simulink model "torqueBalancingSOT_logData"  (Simulink 8.8)
settings: Solver=FixedStepDiscrete  StartTime=0.0  StopTime=CONFIG.SIMULATION_TIME  FixedStep=CONFIG.Ts  RelTol=1e-3  EnableMultiTasking=on
InitFcn:
  | cd(fileparts(which(bdroot)));
  | initTorqueBalancingSOT;
undefined symbols (not defined in the file or in its folder): CONFIG, ConstraintsFeetMatrix, DiscIntNeverNeededParam, gain, reg, ROBOT_DOF, sat, sm, upperBoundFeetConstraints, WBT_robotName
libraries: WBToolboxLibrary x69
(part 1 of 2)
settings Model: SuppressorTable=22 serialization::archive 11 0 3 0 0 0 11 0  Creator=marie  LastModifiedBy=marie
settings DataIOCC: LimitDataPoints=off  SaveFormat=Dataset  SignalLoggingSaveFormat=Dataset
settings DebuggingCC: UnderspecifiedInitializationDetection=Simplified  MergeDetectMultiDrivingBlocksExec=error  FcnCallInpInsideContextMsg=error  StateNameClashWarn=none  SFUnexpectedBacktrackingDiag=error  SFNoUnconditionalDefaultTransitionDiag=error
settings HardwareCC: ProdBitPerPointer=64  ProdBitPerSizeT=64  ProdBitPerPtrDiffT=64  ProdLargestAtomicFloat=Float  ProdIntDivRoundTo=Zero  ProdEndianess=LittleEndian  ProdWordSize=64  ProdHWDeviceType=Intel->x86-64 (Windows64)
settings ModelReferenceCC: PropagateSignalLabelsOutOfModel=on
settings GRTTargetCC: TargetLangStandard=C99 (ISO)  GeneratePreprocessorConditionals=Use local settings  CombineOutputUpdateFcns=on  GRTInterface=off
settings ConfigComp: CovMetricSettings=dwe  CovHtmlReporting=off  CovSaveCumulativeToWorkspaceVar=off  CovSaveSingleToWorkspaceVar=off  CovExternalEMLEnable=on

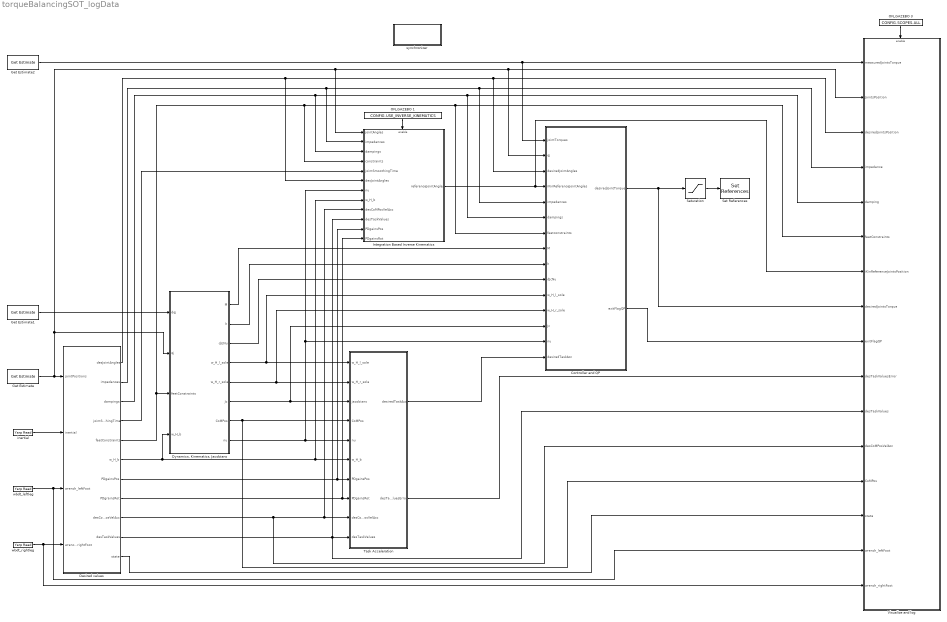
== system torqueBalancingSOT_logData ==
  Controller and QP : Subsystem
  Desired values : Subsystem
  "Dynamics, Kinematics, Jacobians" : Subsystem
  Get Estimate : WBToolboxLibrary/wholeBodyStates/Get Estimate  estimateType=Joints Position  robotName=WBT_robotName  localName=WBT_modelName  wbiFile=WBT_wbiFilename  wbiList=WBT_wbiList
  Get Estimate1 : WBToolboxLibrary/wholeBodyStates/Get Estimate  estimateType=Joints Velocity  robotName=WBT_robotName  localName=WBT_modelName  wbiFile=WBT_wbiFilename  wbiList=WBT_wbiList
  Get Estimate2 : WBToolboxLibrary/wholeBodyStates/Get Estimate  estimateType=Joints Torque  robotName=WBT_robotName  localName=WBT_modelName  wbiFile=WBT_wbiFilename  wbiList=WBT_wbiList
  Integration Based Inverse Kinematics : Subsystem
  ON_GAZEBO 1 : Constant  Value=CONFIG.USE_INVERSE_KINEMATICS
  ON_GAZEBO 3 : Constant  Value=CONFIG.SCOPES.ALL
  Saturation : Saturate  UpperLimit=sat.torque  LowerLimit=-sat.torque
  Set References : WBToolboxLibrary/wholeBodyActuators/Set References  controlType=Torque  fullOrSubControl=Full  controlledJoints=''  robotName=WBT_robotName  localName=WBT_modelName  wbiFile=WBT_wbiFilename  wbiList=WBT_wbiList
  Task Acceleration : Subsystem
  Visualize and log : Subsystem
  inertial : WBToolboxLibrary/Utilities/Yarp Read  portName=PORTS.IMU  signalSize=12  blocking=off  timestamp=off  autoconnect=on  errorOnConnection=on
  synchronizer : Subsystem
      mask Display: disp('SYNCHRONIZER')
  wbdt_leftleg : WBToolboxLibrary/Utilities/Yarp Read  portName=PORTS.WBDT_LEFTLEG_EE  signalSize=6  blocking=off  timestamp=off  autoconnect=on  errorOnConnection=off
  wbdt_rightleg : WBToolboxLibrary/Utilities/Yarp Read  portName=PORTS.WBDT_RIGHTLEG_EE  signalSize=6  blocking=off  timestamp=off  autoconnect=on  errorOnConnection=off
  wires:
  "Dynamics, Kinematics, Jacobians"/7(CoMPos) -> Visualize and log/13(CoMPos), Task Acceleration/4(CoMPos)
  Desired values/9(desCoMPosVelAcc) -> Visualize and log/12(desCoMPosVelAcc), Integration Based Inverse Kinematics/9(desCoMPosVelAcc), Task Acceleration/9(desCoMPosVelAcc)
  "Dynamics, Kinematics, Jacobians"/8(nu) -> Integration Based Inverse Kinematics/7(nu), Controller and QP/14(nu), Task Acceleration/5(nu)
  Desired values/10(desTaskValues) -> Integration Based Inverse Kinematics/10(desTaskValues), Visualize and log/11(desTaskValues), Task Acceleration/10(desTaskValues)
  Desired values/7(PDgainsPos) -> Integration Based Inverse Kinematics/11(PDgainsPos), Task Acceleration/7(PDgainsPos)
  "Dynamics, Kinematics, Jacobians"/5(w_H_r_sole) -> Controller and QP/12(w_H_r_sole), Task Acceleration/2(w_H_r_sole)
  "Dynamics, Kinematics, Jacobians"/4(w_H_l_sole) -> Controller and QP/11(w_H_l_sole), Task Acceleration/1(w_H_l_sole)
  Desired values/2(impedances) -> Integration Based Inverse Kinematics/2(impedances), Visualize and log/4(impedance), Controller and QP/5(impedances)
  "Dynamics, Kinematics, Jacobians"/1(M) -> Controller and QP/8(M)
  "Dynamics, Kinematics, Jacobians"/2(h) -> Controller and QP/9(h)
  Desired values/3(dampings) -> Integration Based Inverse Kinematics/3(dampings), Controller and QP/6(dampings), Visualize and log/5(damping)
  Controller and QP/1(desiredJointTorques) -> Saturation/1, Visualize and log/8(desiredJointsTorque)
  Saturation/1 -> Set References/1
  ON_GAZEBO 3/1 -> Visualize and log/Enable
  Controller and QP/2(exitFlagQP) -> Visualize and log/9(exitFlagQP)
  Task Acceleration/2(desTaskValuesError) -> Visualize and log/10(desTaskValuesError)
  inertial/1 -> Desired values/2(inertial)
  wbdt_leftleg/1 -> Desired values/3(wrench_leftFoot), Visualize and log/15(wrench_leftFoot)
  wbdt_rightleg/1 -> Desired values/4(wrench_rightFoot), Visualize and log/16(wrench_rightFoot)
  Get Estimate1/1 -> "Dynamics, Kinematics, Jacobians"/1(dqj)
  Get Estimate2/1 -> Visualize and log/1(measuredJointsTorque), Controller and QP/1(jointTorques)
  Desired values/6(w_H_b) -> "Dynamics, Kinematics, Jacobians"/4(w_H_b), Integration Based Inverse Kinematics/8(w_H_b), Task Acceleration/6(w_H_b)
  Get Estimate/1 -> Visualize and log/2(JointsPosition), Controller and QP/2(qj), Integration Based Inverse Kinematics/1(jointAngles), "Dynamics, Kinematics, Jacobians"/2(qj), Desired values/1(jointPositions)
  "Dynamics, Kinematics, Jacobians"/6(Jc) -> Controller and QP/13(Jc), Task Acceleration/3(jacobians)
  Desired values/5(feetConstraints) -> Controller and QP/7(feetconstraints), Visualize and log/6(feetConstraints), Integration Based Inverse Kinematics/4(constraints), "Dynamics, Kinematics, Jacobians"/3(feetConstraints)
  "Dynamics, Kinematics, Jacobians"/3(dJcNu) -> Controller and QP/10(dJcNu)
  Task Acceleration/1(desiredTaskAcc) -> Controller and QP/15(desiredTaskAcc)
  Desired values/11(state) -> Visualize and log/14(state)
  Integration Based Inverse Kinematics/1(referenceJointAngles) -> Visualize and log/7(iKinReferenceJointsPosition), Controller and QP/4(iKinReferenceJointAngles)
  Desired values/1(desJointAngles) -> Integration Based Inverse Kinematics/6(desJointAngles), Visualize and log/3(desiredJointsPosition), Controller and QP/3(desiredJointAngles)
  ON_GAZEBO 1/1 -> Integration Based Inverse Kinematics/Enable
  Desired values/8(PDgrainsRot) -> Integration Based Inverse Kinematics/12(PDgainsRot), Task Acceleration/8(PDgainsRot)
  Desired values/4(jointSmoothingTime) -> Integration Based Inverse Kinematics/5(jointSmoothingTime)

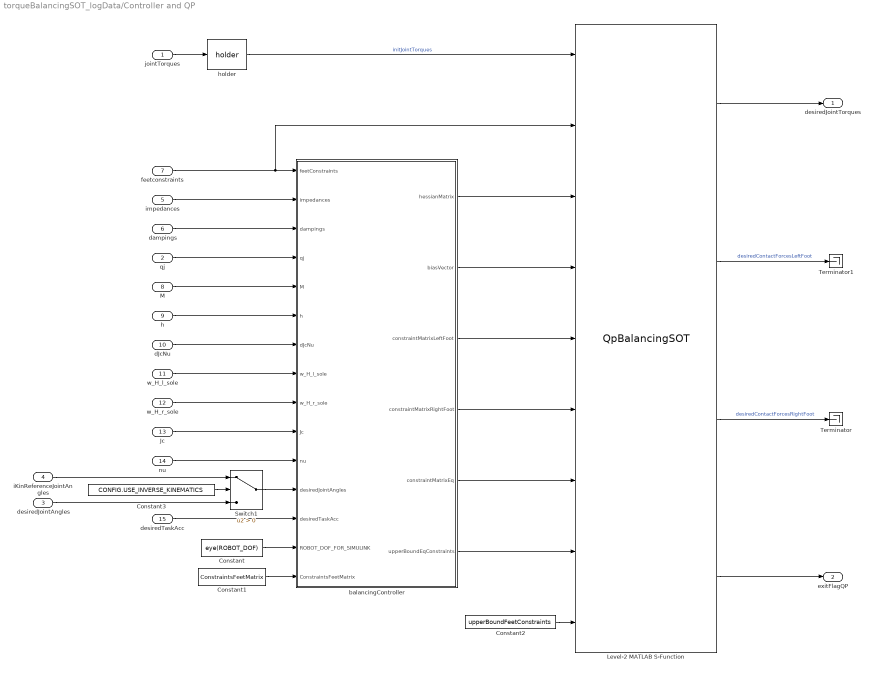
== system torqueBalancingSOT_logData/Controller and QP ==
  jointTorques : Inport
  qj : Inport  Port=2
  desiredJointAngles : Inport  Port=3
  iKinReferenceJointAngles : Inport  Port=4
  impedances : Inport  Port=5
  dampings : Inport  Port=6
  feetconstraints : Inport  Port=7
  M : Inport  Port=8
  h : Inport  Port=9
  dJcNu : Inport  Port=10
  w_H_l_sole : Inport  Port=11
  w_H_r_sole : Inport  Port=12
  Jc : Inport  Port=13
  nu : Inport  Port=14
  desiredTaskAcc : Inport  Port=15
  Constant : Constant  Value=eye(ROBOT_DOF)
  Constant1 : Constant  Value=ConstraintsFeetMatrix
  Constant2 : Constant  Value=upperBoundFeetConstraints
  Constant3 : Constant  Value=CONFIG.USE_INVERSE_KINEMATICS
  Level-2 MATLAB S-Function : M-S-Function  FunctionName=QpBalancingSOT  Parameters=ROBOT_DOF,sat.torqueDot,CONFIG.Ts,CONFIG.QP.USE_CONTINUITY_CONSTRAINTS,CONFIG.QP.USE_STRICT_TASK_PRIORITIES  mask{robotDofs=ROBOT_DOF, tauDotMax=sat.torqueDot, Ts=CONFIG.Ts}
      mask prompts: robotDofs "Robt degrees of freedom"; tauDotMax "Maximum derivative of torques"; Ts "Controller period"
      mask Display: disp('QP')
  Switch1 : Switch  Criteria=u2 > Threshold
  Terminator : Terminator
  Terminator1 : Terminator
  balancingController : MATLAB Function  TreatAsAtomicUnit=on
  "holder " : WBToolboxLibrary/Utilities/holder 
  desiredJointTorques : Outport
  exitFlagQP : Outport  Port=2
  wires:
  balancingController/1(hessianMatrix) -> Level-2 MATLAB S-Function/3
  feetconstraints/1 -> Level-2 MATLAB S-Function/2, balancingController/1(feetConstraints)
  qj/1 -> balancingController/4(qj)
  impedances/1 -> balancingController/2(impedances)
  M/1 -> balancingController/5(M)
  h/1 -> balancingController/6(h)
  dJcNu/1 -> balancingController/7(dJcNu)
  w_H_l_sole/1 -> balancingController/8(w_H_l_sole)
  w_H_r_sole/1 -> balancingController/9(w_H_r_sole)
  Jc/1 -> balancingController/10(Jc)
  nu/1 -> balancingController/11(nu)
  desiredTaskAcc/1 -> balancingController/13(desiredTaskAcc)
  Constant/1 -> balancingController/14(ROBOT_DOF_FOR_SIMULINK)
  Constant1/1 -> balancingController/15(ConstraintsFeetMatrix)
  dampings/1 -> balancingController/3(dampings)
  balancingController/2(biasVector) -> Level-2 MATLAB S-Function/4
  balancingController/3(constraintMatrixLeftFoot) -> Level-2 MATLAB S-Function/5
  balancingController/4(constraintMatrixRightFoot) -> Level-2 MATLAB S-Function/6
  balancingController/5(constraintMatrixEq) -> Level-2 MATLAB S-Function/7
  balancingController/6(upperBoundEqConstraints) -> Level-2 MATLAB S-Function/8
  Constant2/1 -> Level-2 MATLAB S-Function/9
  Level-2 MATLAB S-Function/1 -> desiredJointTorques/1
  Level-2 MATLAB S-Function/2 -> Terminator1/1  "desiredContactForcesLeftFoot"
  Level-2 MATLAB S-Function/3 -> Terminator/1  "desiredContactForcesRightFoot"
  Level-2 MATLAB S-Function/4 -> exitFlagQP/1
  jointTorques/1 -> "holder "/1
  "holder "/1 -> Level-2 MATLAB S-Function/1  "initJointTorques"
  Constant3/1 -> Switch1/2
  iKinReferenceJointAngles/1 -> Switch1/1
  desiredJointAngles/1 -> Switch1/3
  Switch1/1 -> balancingController/12(desiredJointAngles)

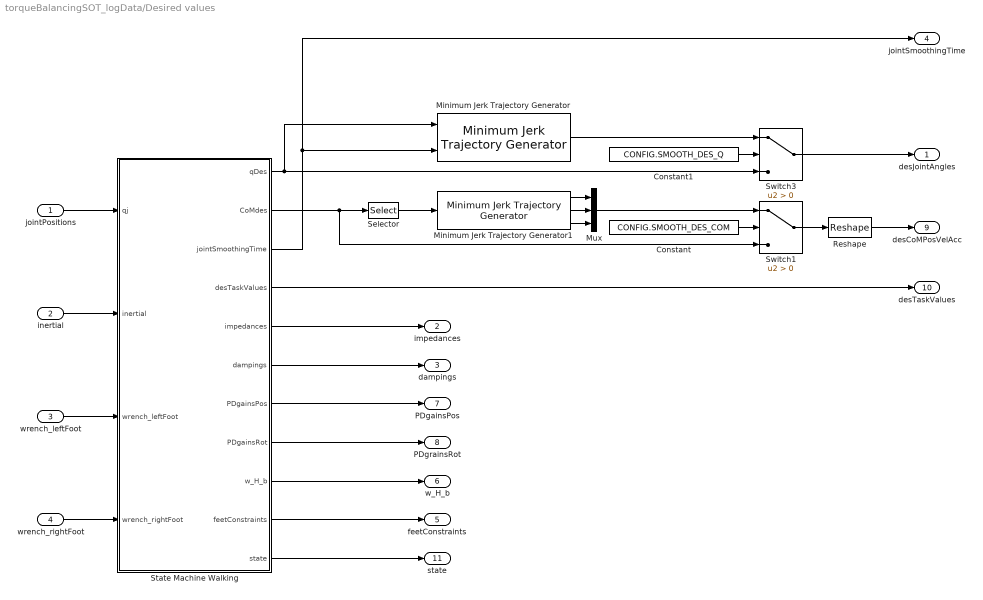
== system torqueBalancingSOT_logData/Desired values ==
  jointPositions : Inport
  inertial : Inport  Port=2
  wrench_leftFoot : Inport  Port=3
  wrench_rightFoot : Inport  Port=4
  Constant : Constant  Value=CONFIG.SMOOTH_DES_COM
  Constant1 : Constant  Value=CONFIG.SMOOTH_DES_Q
  Minimum Jerk Trajectory Generator : WBToolboxLibrary/Utilities/Minimum Jerk Trajectory Generator  externalSettlingTime=on  settlingTime=3  sampleTime=CONFIG.Ts  resetOnSettlingTime=off  firstDerivatives=off  secondDerivatives=off  explicitInitialValue=off
  Minimum Jerk Trajectory Generator1 : WBToolboxLibrary/Utilities/Minimum Jerk Trajectory Generator  externalSettlingTime=off  settlingTime=gain.SmoothingTimeTasks  sampleTime=CONFIG.Ts  resetOnSettlingTime=off  firstDerivatives=on  secondDerivatives=on  explicitInitialValue=off
  Mux : Mux  Inputs=3
  Reshape : Reshape  OutputDimensionality=Customize  OutputDimensions=[3,3]
  Selector : Selector  InputPortWidth=9  IndexOptions=Index vector (dialog)  Indices=[1 2 3]  OutputSizes=1
  State Machine Walking : Subsystem
  Switch1 : Switch  Criteria=u2 > Threshold
  Switch3 : Switch  Criteria=u2 > Threshold
  desJointAngles : Outport
  impedances : Outport  Port=2
  dampings : Outport  Port=3
  jointSmoothingTime : Outport  Port=4
  feetConstraints : Outport  Port=5
  w_H_b : Outport  Port=6
  PDgainsPos : Outport  Port=7
  PDgrainsRot : Outport  Port=8
  desCoMPosVelAcc : Outport  Port=9
  desTaskValues : Outport  Port=10
  state : Outport  Port=11
  wires:
  Constant/1 -> Switch1/2
  Constant1/1 -> Switch3/2
  Minimum Jerk Trajectory Generator1/3 -> Mux/3
  Minimum Jerk Trajectory Generator1/2 -> Mux/2
  State Machine Walking/7(PDgainsPos) -> PDgainsPos/1
  State Machine Walking/9(w_H_b) -> w_H_b/1
  State Machine Walking/11(state) -> state/1
  Mux/1 -> Switch1/1
  Minimum Jerk Trajectory Generator1/1 -> Mux/1
  State Machine Walking/5(impedances) -> impedances/1
  Selector/1 -> Minimum Jerk Trajectory Generator1/1
  State Machine Walking/3(jointSmoothingTime) -> jointSmoothingTime/1, Minimum Jerk Trajectory Generator/2
  Switch1/1 -> Reshape/1
  Switch3/1 -> desJointAngles/1
  State Machine Walking/2(CoMdes) -> Switch1/3, Selector/1
  State Machine Walking/4(desTaskValues) -> desTaskValues/1
  State Machine Walking/10(feetConstraints) -> feetConstraints/1
  State Machine Walking/1(qDes) -> Minimum Jerk Trajectory Generator/1, Switch3/3
  Reshape/1 -> desCoMPosVelAcc/1
  jointPositions/1 -> State Machine Walking/1(qj)
  State Machine Walking/6(dampings) -> dampings/1
  wrench_rightFoot/1 -> State Machine Walking/4(wrench_rightFoot)
  wrench_leftFoot/1 -> State Machine Walking/3(wrench_leftFoot)
  inertial/1 -> State Machine Walking/2(inertial)
  State Machine Walking/8(PDgainsRot) -> PDgrainsRot/1
  Minimum Jerk Trajectory Generator/1 -> Switch3/1

== system torqueBalancingSOT_logData/Dynamics, Kinematics, Jacobians ==
  dqj : Inport
  qj : Inport  Port=2
  feetConstraints : Inport  Port=3
  w_H_b : Inport  Port=4
  CoM/Base Kinematics : Subsystem
  Jacobians : Subsystem
  System Dynamics : Subsystem
  M : Outport
  h : Outport  Port=2
  dJcNu : Outport  Port=3
  w_H_l_sole : Outport  Port=4
  w_H_r_sole : Outport  Port=5
  Jc : Outport  Port=6
  CoMPos : Outport  Port=7
  nu : Outport  Port=8
  wires:
  qj/1 -> Jacobians/4(qj), System Dynamics/3(qj), CoM/Base Kinematics/2(qj)
  w_H_b/1 -> Jacobians/3(w_H_b), System Dynamics/2(w_H_b), CoM/Base Kinematics/1(w_H_b)
  CoM/Base Kinematics/1(CoMPos) -> CoMPos/1
  Jacobians/1(Jc) -> Jc/1
  Jacobians/2(dJcNu) -> dJcNu/1
  System Dynamics/2(M) -> M/1
  System Dynamics/1(h) -> h/1
  CoM/Base Kinematics/2(w_H_l_sole) -> w_H_l_sole/1
  CoM/Base Kinematics/3(w_H_r_sole) -> w_H_r_sole/1
  dqj/1 -> Jacobians/2(dqj)
  feetConstraints/1 -> Jacobians/1(feetConstraints)
  Jacobians/3(nu) -> nu/1, System Dynamics/1(nu)

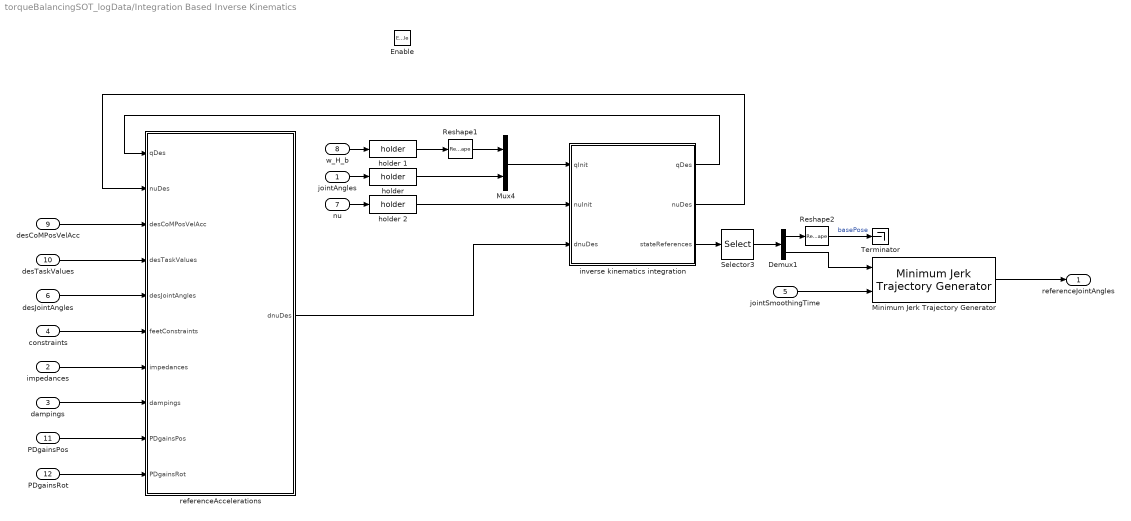
== system torqueBalancingSOT_logData/Integration Based Inverse Kinematics ==
  jointAngles : Inport
  impedances : Inport  Port=2
  dampings : Inport  Port=3
  constraints : Inport  Port=4
  jointSmoothingTime : Inport  Port=5
  desJointAngles : Inport  Port=6
  nu : Inport  Port=7
  w_H_b : Inport  Port=8
  desCoMPosVelAcc : Inport  Port=9
  desTaskValues : Inport  Port=10
  PDgainsPos : Inport  Port=11
  PDgainsRot : Inport  Port=12
  Enable : EnablePort
  Demux1 : Demux  Outputs=[16,ROBOT_DOF]
  Minimum Jerk Trajectory Generator : WBToolboxLibrary/Utilities/Minimum Jerk Trajectory Generator  externalSettlingTime=on  settlingTime=0.5  sampleTime=CONFIG.Ts  resetOnSettlingTime=off  firstDerivatives=off  secondDerivatives=off  explicitInitialValue=off
  Mux4 : Mux  Inputs=2
  Reshape1 : Reshape
  Reshape2 : Reshape  OutputDimensionality=Customize  OutputDimensions=[4,4]
  Selector3 : Selector  NumberOfDimensions=2  InputPortWidth=3  IndexOptions=Index vector (dialog),Index vector (dialog)  Indices=[1:(ROBOT_DOF+16)],[1]  OutputSizes=1,1
  Terminator : Terminator
  "holder " : WBToolboxLibrary/Utilities/holder 
  holder 1 : WBToolboxLibrary/Utilities/holder 
  holder 2 : WBToolboxLibrary/Utilities/holder 
  inverse kinematics integration : Subsystem
  referenceAccelerations : Subsystem
  referenceJointAngles : Outport
  wires:
  Mux4/1 -> inverse kinematics integration/1(qInit)
  desCoMPosVelAcc/1 -> referenceAccelerations/3(desCoMPosVelAcc)
  constraints/1 -> referenceAccelerations/6(feetConstraints)
  holder 1/1 -> Reshape1/1
  Reshape1/1 -> Mux4/1
  "holder "/1 -> Mux4/2
  jointAngles/1 -> "holder "/1
  w_H_b/1 -> holder 1/1
  desJointAngles/1 -> referenceAccelerations/5(desJointAngles)
  desTaskValues/1 -> referenceAccelerations/4(desTaskValues)
  holder 2/1 -> inverse kinematics integration/2(nuInit)
  referenceAccelerations/1(dnuDes) -> inverse kinematics integration/3(dnuDes)
  inverse kinematics integration/1(qDes) -> referenceAccelerations/1(qDes)
  inverse kinematics integration/2(nuDes) -> referenceAccelerations/2(nuDes)
  inverse kinematics integration/3(stateReferences) -> Selector3/1
  nu/1 -> holder 2/1
  Selector3/1 -> Demux1/1
  Reshape2/1 -> Terminator/1  "basePose"
  Demux1/1 -> Reshape2/1
  Demux1/2 -> Minimum Jerk Trajectory Generator/1
  Minimum Jerk Trajectory Generator/1 -> referenceJointAngles/1
  impedances/1 -> referenceAccelerations/7(impedances)
  dampings/1 -> referenceAccelerations/8(dampings)
  PDgainsPos/1 -> referenceAccelerations/9(PDgainsPos)
  PDgainsRot/1 -> referenceAccelerations/10(PDgainsRot)
  jointSmoothingTime/1 -> Minimum Jerk Trajectory Generator/2

== system torqueBalancingSOT_logData/Task Acceleration ==
  w_H_l_sole : Inport
  w_H_r_sole : Inport  Port=2
  jacobians : Inport  Port=3
  CoMPos : Inport  Port=4
  nu : Inport  Port=5
  w_H_b : Inport  Port=6
  PDgainsPos : Inport  Port=7
  PDgainsRot : Inport  Port=8
  desCoMPosVelAcc : Inport  Port=9
  desTaskValues : Inport  Port=10
  Bus Creator : BusCreator  Inputs='rootRotError','leftFootOriginError','leftFootRotError','rightFootOriginError','rightFootRotError'
  Bus Selector : BusSelector  OutputSignals=desRootRotPosVelAcc,desLeftFootOriginPosVelAcc,desLeftFootRotPosVelAcc,desRightFootOriginPosVelAcc,desRightFootRotPosVelAcc
  Product : Product  Multiplication=Matrix(*)
  Reshape : Reshape  OutputDimensionality=Customize  OutputDimensions=[3,2]
  Reshape1 : Reshape  OutputDimensionality=Customize  OutputDimensions=[1,18]
  Selector1 : Selector  NumberOfDimensions=2  InputPortWidth=9  IndexOptions=Index vector (dialog),Index vector (dialog)  Indices=[1:3],[1:3]  OutputSizes=1,1
  desiredTaskAcceleration : MATLAB Function  TreatAsAtomicUnit=on
  desiredTaskAcc : Outport
  desTaskValuesError : Outport  Port=2
  wires:
  Bus Selector/1 -> desiredTaskAcceleration/7(desRootRotPosVelAcc)  "<desRootRotPosVelAcc>"
  Bus Selector/2 -> desiredTaskAcceleration/8(desLeftFootOriginPosVelAcc)  "<desLeftFootOriginPosVelAcc>"
  Bus Selector/3 -> desiredTaskAcceleration/9(desLeftFootRotPosVelAcc)  "<desLeftFootRotPosVelAcc>"
  Bus Selector/4 -> desiredTaskAcceleration/10(desRightFootOriginPosVelAcc)  "<desRightFootOriginPosVelAcc>"
  desTaskValues/1 -> Bus Selector/1
  w_H_b/1 -> Selector1/1
  Bus Selector/5 -> desiredTaskAcceleration/11(desRightFootRotPosVelAcc)  "<desRightFootRotPosVelAcc>"
  jacobians/1 -> Product/1
  nu/1 -> Product/2
  CoMPos/1 -> desiredTaskAcceleration/4(CoMPos)
  desCoMPosVelAcc/1 -> desiredTaskAcceleration/6(desCoMPosVelAcc)
  Product/1 -> desiredTaskAcceleration/3(taskVelocities)
  desiredTaskAcceleration/2(rootRotError) -> Bus Creator/1
  desiredTaskAcceleration/3(leftFootOriginError) -> Bus Creator/2
  desiredTaskAcceleration/4(leftFootRotError) -> Bus Creator/3
  desiredTaskAcceleration/5(rightFootOriginError) -> Bus Creator/4
  desiredTaskAcceleration/6(rightFootRotError) -> Bus Creator/5
  desiredTaskAcceleration/1(desiredTaskAcc) -> desiredTaskAcc/1
  Bus Creator/1 -> desTaskValuesError/1
  w_H_r_sole/1 -> desiredTaskAcceleration/2(w_H_r_sole)
  w_H_l_sole/1 -> desiredTaskAcceleration/1(w_H_l_sole)
  Selector1/1 -> desiredTaskAcceleration/5(fixedLink_R_root)
  PDgainsRot/1 -> Reshape/1
  Reshape/1 -> desiredTaskAcceleration/13(PDgainsRot)
  PDgainsPos/1 -> Reshape1/1
  Reshape1/1 -> desiredTaskAcceleration/12(PDgainsPos)

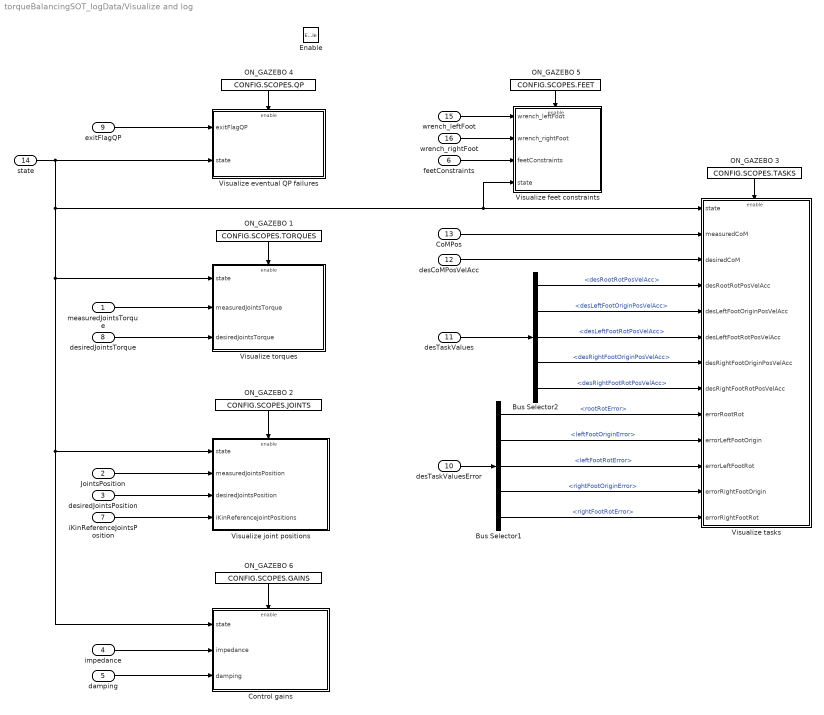
== system torqueBalancingSOT_logData/Visualize and log ==
  measuredJointsTorque : Inport
  JointsPosition : Inport  Port=2
  desiredJointsPosition : Inport  Port=3
  impedance : Inport  Port=4
  damping : Inport  Port=5
  feetConstraints : Inport  Port=6
  iKinReferenceJointsPosition : Inport  Port=7
  desiredJointsTorque : Inport  Port=8
  exitFlagQP : Inport  Port=9
  desTaskValuesError : Inport  Port=10
  desTaskValues : Inport  Port=11
  desCoMPosVelAcc : Inport  Port=12
  CoMPos : Inport  Port=13
  state : Inport  Port=14
  wrench_leftFoot : Inport  Port=15
  wrench_rightFoot : Inport  Port=16
  Enable : EnablePort
  Bus Selector1 : BusSelector  OutputSignals=rootRotError,leftFootOriginError,leftFootRotError,rightFootOriginError,rightFootRotError
  Bus Selector2 : BusSelector  OutputSignals=desRootRotPosVelAcc,desLeftFootOriginPosVelAcc,desLeftFootRotPosVelAcc,desRightFootOriginPosVelAcc,desRightFootRotPosVelAcc
  Control gains : Subsystem
  ON_GAZEBO 1 : Constant  Value=CONFIG.SCOPES.TORQUES
  ON_GAZEBO 2 : Constant  Value=CONFIG.SCOPES.JOINTS
  ON_GAZEBO 3 : Constant  Value=CONFIG.SCOPES.TASKS
  ON_GAZEBO 4 : Constant  Value=CONFIG.SCOPES.QP
  ON_GAZEBO 5 : Constant  Value=CONFIG.SCOPES.FEET
  ON_GAZEBO 6 : Constant  Value=CONFIG.SCOPES.GAINS
  Visualize eventual QP failures : Subsystem
  Visualize feet constraints : Subsystem
  Visualize joint positions : Subsystem
  Visualize tasks : Subsystem
  Visualize torques : Subsystem
  wires:
  ON_GAZEBO 4/1 -> Visualize eventual QP failures/Enable
  exitFlagQP/1 -> Visualize eventual QP failures/1(exitFlagQP)
  measuredJointsTorque/1 -> Visualize torques/2(measuredJointsTorque)
  desiredJointsTorque/1 -> Visualize torques/3(desiredJointsTorque)
  ON_GAZEBO 1/1 -> Visualize torques/Enable
  state/1 -> Visualize eventual QP failures/2(state), Control gains/1(state), Visualize joint positions/1(state), Visualize torques/1(state), Visualize feet constraints/4(state), Visualize tasks/1(state)
  JointsPosition/1 -> Visualize joint positions/2(measuredJointsPosition)
  desiredJointsPosition/1 -> Visualize joint positions/3(desiredJointsPosition)
  ON_GAZEBO 2/1 -> Visualize joint positions/Enable
  CoMPos/1 -> Visualize tasks/2(measuredCoM)
  desCoMPosVelAcc/1 -> Visualize tasks/3(desiredCoM)
  Bus Selector2/3 -> Visualize tasks/6(desLeftFootRotPosVelAcc)  "<desLeftFootRotPosVelAcc>"
  Bus Selector2/2 -> Visualize tasks/5(desLeftFootOriginPosVelAcc)  "<desLeftFootOriginPosVelAcc>"
  Bus Selector2/5 -> Visualize tasks/8(desRightFootRotPosVelAcc)  "<desRightFootRotPosVelAcc>"
  Bus Selector2/4 -> Visualize tasks/7(desRightFootOriginPosVelAcc)  "<desRightFootOriginPosVelAcc>"
  desTaskValues/1 -> Bus Selector2/1
  Bus Selector2/1 -> Visualize tasks/4(desRootRotPosVelAcc)  "<desRootRotPosVelAcc>"
  desTaskValuesError/1 -> Bus Selector1/1
  Bus Selector1/1 -> Visualize tasks/9(errorRootRot)  "<rootRotError>"
  Bus Selector1/2 -> Visualize tasks/10(errorLeftFootOrigin)  "<leftFootOriginError>"
  Bus Selector1/3 -> Visualize tasks/11(errorLeftFootRot)  "<leftFootRotError>"
  Bus Selector1/4 -> Visualize tasks/12(errorRightFootOrigin)  "<rightFootOriginError>"
  Bus Selector1/5 -> Visualize tasks/13(errorRightFootRot)  "<rightFootRotError>"
  ON_GAZEBO 3/1 -> Visualize tasks/Enable
  feetConstraints/1 -> Visualize feet constraints/3(feetConstraints)
  ON_GAZEBO 5/1 -> Visualize feet constraints/Enable
  wrench_rightFoot/1 -> Visualize feet constraints/2(wrench_rightFoot)
  wrench_leftFoot/1 -> Visualize feet constraints/1(wrench_leftFoot)
  impedance/1 -> Control gains/2(impedance)
  damping/1 -> Control gains/3(damping)
  ON_GAZEBO 6/1 -> Control gains/Enable
  iKinReferenceJointsPosition/1 -> Visualize joint positions/4(iKinReferenceJointPositions)

== system torqueBalancingSOT_logData/synchronizer ==
  GAZEBO_SYNCHRONIZER : Subsystem
  Logical Operator : Logic  Operator=NOT  AllPortsSameDT=off  OutDataTypeStr=boolean
  "ON_GAZEBO " : Constant  Value=CONFIG.ON_GAZEBO
  REAL_TIME_SYNC : Subsystem
  wires:
  Logical Operator/1 -> REAL_TIME_SYNC/Enable
  "ON_GAZEBO "/1 -> GAZEBO_SYNCHRONIZER/Enable, Logical Operator/1

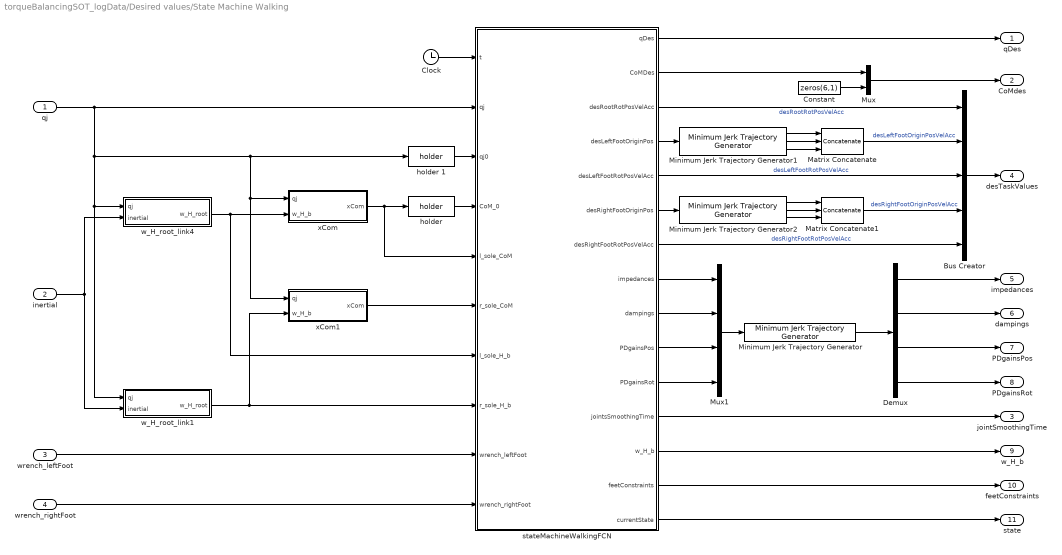
== system torqueBalancingSOT_logData/Desired values/State Machine Walking ==
  qj : Inport
  inertial : Inport  Port=2
  wrench_leftFoot : Inport  Port=3
  wrench_rightFoot : Inport  Port=4
  Bus Creator : BusCreator  Inputs='desRootRotPosVelAcc','desLeftFootOriginPosVelAcc','desLeftFootRotPosVelAcc','desRightFootOriginPosVelAcc','desRightFootRotPosVelAcc'
  Clock : Clock
  Constant : Constant  Value=zeros(6,1)
  Demux : Demux  Outputs=[ROBOT_DOF, ROBOT_DOF, 18, 6]
  Matrix Concatenate : Concatenate  NumInputs=3  Mode=Multidimensional array  ConcatenateDimension=2
  Matrix Concatenate1 : Concatenate  NumInputs=3  Mode=Multidimensional array  ConcatenateDimension=2
  Minimum Jerk Trajectory Generator : WBToolboxLibrary/Utilities/Minimum Jerk Trajectory Generator  externalSettlingTime=off  settlingTime=gain.SmoothingTimeGainScheduling  sampleTime=CONFIG.Ts  resetOnSettlingTime=off  firstDerivatives=off  secondDerivatives=off  explicitInitialValue=off
  Minimum Jerk Trajectory Generator1 : WBToolboxLibrary/Utilities/Minimum Jerk Trajectory Generator  externalSettlingTime=off  settlingTime=gain.SmoothingTimeTasks  sampleTime=CONFIG.Ts  resetOnSettlingTime=off  firstDerivatives=on  secondDerivatives=on  explicitInitialValue=off
  Minimum Jerk Trajectory Generator2 : WBToolboxLibrary/Utilities/Minimum Jerk Trajectory Generator  externalSettlingTime=off  settlingTime=gain.SmoothingTimeTasks  sampleTime=CONFIG.Ts  resetOnSettlingTime=off  firstDerivatives=on  secondDerivatives=on  explicitInitialValue=off
  Mux : Mux  Inputs=2
  Mux1 : Mux
  "holder " : WBToolboxLibrary/Utilities/holder 
  holder 1 : WBToolboxLibrary/Utilities/holder 
  stateMachineWalkingFCN : MATLAB Function  TreatAsAtomicUnit=on
  w_H_root_link1 : Subsystem  mask{link_name='r_sole'}
      mask prompts: link_name "link name"
      mask help:
      | This block evaluates the homogeneous transformation between the world and the root link, i.e. ^wH_b. It assumes that the link specified by the variable 'link_name' has a constant position
      | w.r.t. an inertial frame, but it can rotate arbitrarily. This rotation is retrived from the IMU sensor.
      mask Display:
      | str = strrep(link_name, '_','\_');
      | port_label('output',1,['{}^{',str '}H_{root}'],'texmode','on')
      | clear str;
      | 
      | port_label('input',1,'q_j','texmode','on')
      | 
      | port_label('input',2,'inertial','texmode','on')
  w_H_root_link4 : Subsystem  mask{link_name='l_sole'}
      mask prompts: link_name "link name"
      mask help:
      | This block evaluates the homogeneous transformation between the world and the root link, i.e. ^wH_b. It assumes that the link specified by the variable 'link_name' has a constant position
      | w.r.t. an inertial frame, but it can rotate arbitrarily. This rotation is retrived from the IMU sensor.
      mask Display:
      | str = strrep(link_name, '_','\_');
      | port_label('output',1,['{}^{',str '}H_{root}'],'texmode','on')
      | clear str;
      | 
      | port_label('input',1,'q_j','texmode','on')
      | 
      | port_label('input',2,'inertial','texmode','on')
  xCom : Subsystem
  xCom1 : Subsystem
  qDes : Outport
  CoMdes : Outport  Port=2
  jointSmoothingTime : Outport  Port=3
  desTaskValues : Outport  Port=4
  impedances : Outport  Port=5
  dampings : Outport  Port=6
  PDgainsPos : Outport  Port=7
  PDgainsRot : Outport  Port=8
  w_H_b : Outport  Port=9
  feetConstraints : Outport  Port=10
  state : Outport  Port=11
  wires:
  Clock/1 -> stateMachineWalkingFCN/1(t)
  stateMachineWalkingFCN/8(impedances) -> Mux1/1
  stateMachineWalkingFCN/7(desRightFootRotPosVelAcc) -> Bus Creator/5  "desRightFootRotPosVelAcc"
  Bus Creator/1 -> desTaskValues/1
  wrench_rightFoot/1 -> stateMachineWalkingFCN/10(wrench_rightFoot)
  stateMachineWalkingFCN/13(w_H_b) -> w_H_b/1
  wrench_leftFoot/1 -> stateMachineWalkingFCN/9(wrench_leftFoot)
  Mux1/1 -> Minimum Jerk Trajectory Generator/1
  qj/1 -> w_H_root_link1/1(qj), w_H_root_link4/1(qj), xCom1/1(qj), xCom/1(qj), holder 1/1, stateMachineWalkingFCN/2(qj)
  holder 1/1 -> stateMachineWalkingFCN/3(qj0)
  xCom1/1(xCom) -> stateMachineWalkingFCN/6(r_sole_CoM)
  "holder "/1 -> stateMachineWalkingFCN/4(CoM_0)
  w_H_root_link4/1(w_H_root) -> stateMachineWalkingFCN/7(l_sole_H_b), xCom/2(w_H_b)
  inertial/1 -> w_H_root_link4/2(inertial), w_H_root_link1/2(inertial)
  xCom/1(xCom) -> "holder "/1, stateMachineWalkingFCN/5(l_sole_CoM)
  Minimum Jerk Trajectory Generator/1 -> Demux/1
  stateMachineWalkingFCN/14(feetConstraints) -> feetConstraints/1
  stateMachineWalkingFCN/2(CoMDes) -> Mux/1
  w_H_root_link1/1(w_H_root) -> stateMachineWalkingFCN/8(r_sole_H_b), xCom1/2(w_H_b)
  Demux/1 -> impedances/1
  stateMachineWalkingFCN/12(jointsSmoothingTime) -> jointSmoothingTime/1
  stateMachineWalkingFCN/15(currentState) -> state/1
  stateMachineWalkingFCN/1(qDes) -> qDes/1
  Minimum Jerk Trajectory Generator1/1 -> Matrix Concatenate/1
  Minimum Jerk Trajectory Generator1/2 -> Matrix Concatenate/2
  Minimum Jerk Trajectory Generator1/3 -> Matrix Concatenate/3
  Matrix Concatenate/1 -> Bus Creator/2  "desLeftFootOriginPosVelAcc"
  stateMachineWalkingFCN/4(desLeftFootOriginPos) -> Minimum Jerk Trajectory Generator1/1
  Minimum Jerk Trajectory Generator2/1 -> Matrix Concatenate1/1
  Minimum Jerk Trajectory Generator2/2 -> Matrix Concatenate1/2
  Minimum Jerk Trajectory Generator2/3 -> Matrix Concatenate1/3
  stateMachineWalkingFCN/6(desRightFootOriginPos) -> Minimum Jerk Trajectory Generator2/1
  Matrix Concatenate1/1 -> Bus Creator/4  "desRightFootOriginPosVelAcc"
  stateMachineWalkingFCN/3(desRootRotPosVelAcc) -> Bus Creator/1  "desRootRotPosVelAcc"
  stateMachineWalkingFCN/5(desLeftFootRotPosVelAcc) -> Bus Creator/3  "desLeftFootRotPosVelAcc"
  Demux/3 -> PDgainsPos/1
  Constant/1 -> Mux/2
  Mux/1 -> CoMdes/1
  stateMachineWalkingFCN/9(dampings) -> Mux1/2
  Demux/2 -> dampings/1
  stateMachineWalkingFCN/11(PDgainsRot) -> Mux1/4
  Demux/4 -> PDgainsRot/1
  stateMachineWalkingFCN/10(PDgainsPos) -> Mux1/3

== system torqueBalancingSOT_logData/Dynamics, Kinematics, Jacobians/CoM/Base Kinematics ==
  w_H_b : Inport
  qj : Inport  Port=2
  Forward Kinematics : WBToolboxLibrary/wholeBodyModel/Kinematics/Forward Kinematics  frameName='com'  robotName=WBT_robotName  localName=WBT_modelName  wbiFile=WBT_wbiFilename  wbiList=WBT_wbiList
  Forward Kinematics1 : WBToolboxLibrary/wholeBodyModel/Kinematics/Forward Kinematics  frameName='l_sole'  robotName=WBT_robotName  localName=WBT_modelName  wbiFile=WBT_wbiFilename  wbiList=WBT_wbiList
  Forward Kinematics2 : WBToolboxLibrary/wholeBodyModel/Kinematics/Forward Kinematics  frameName='r_sole'  robotName=WBT_robotName  localName=WBT_modelName  wbiFile=WBT_wbiFilename  wbiList=WBT_wbiList
  Selector : Selector  NumberOfDimensions=2  InputPortWidth=6+ROBOT_DOF  IndexOptions=Index vector (dialog),Index vector (dialog)  Indices=[1:3],[4]  OutputSizes=1,1
  CoMPos : Outport
  w_H_l_sole : Outport  Port=2
  w_H_r_sole : Outport  Port=3
  wires:
  Selector/1 -> CoMPos/1
  qj/1 -> Forward Kinematics1/2, Forward Kinematics2/2, Forward Kinematics/2
  Forward Kinematics/1 -> Selector/1
  w_H_b/1 -> Forward Kinematics1/1, Forward Kinematics2/1, Forward Kinematics/1
  Forward Kinematics2/1 -> w_H_r_sole/1
  Forward Kinematics1/1 -> w_H_l_sole/1

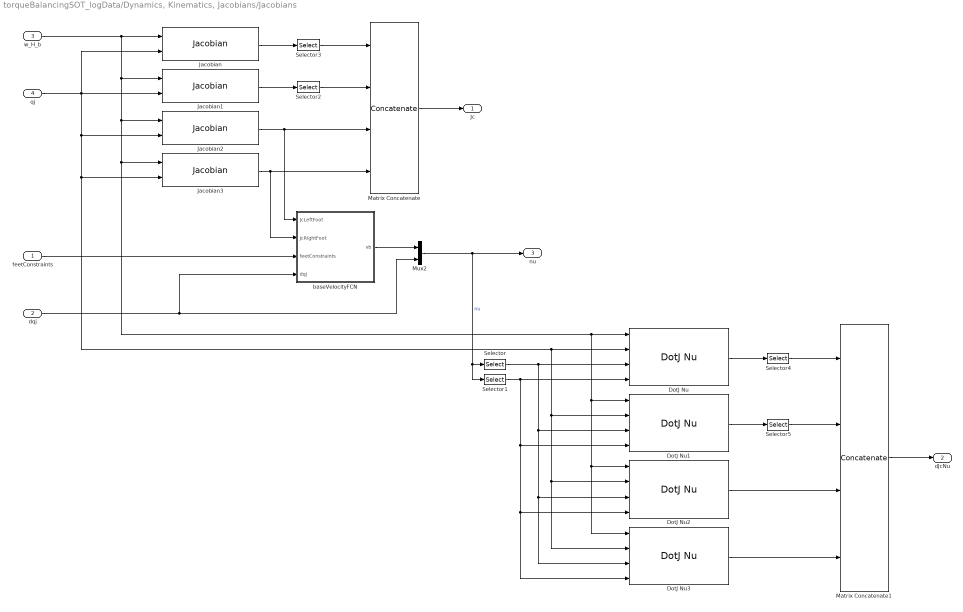
== system torqueBalancingSOT_logData/Dynamics, Kinematics, Jacobians/Jacobians ==
  feetConstraints : Inport
  dqj : Inport  Port=2
  w_H_b : Inport  Port=3
  qj : Inport  Port=4
  DotJ Nu : WBToolboxLibrary/wholeBodyModel/Jacobians/DotJ Nu  frameName='com'  robotName=WBT_robotName  localName=WBT_modelName  wbiFile=WBT_wbiFilename  wbiList=WBT_wbiList
  DotJ Nu1 : WBToolboxLibrary/wholeBodyModel/Jacobians/DotJ Nu  frameName='root_link'  robotName=WBT_robotName  localName=WBT_modelName  wbiFile=WBT_wbiFilename  wbiList=WBT_wbiList
  DotJ Nu2 : WBToolboxLibrary/wholeBodyModel/Jacobians/DotJ Nu  frameName='l_sole'  robotName=WBT_robotName  localName=WBT_modelName  wbiFile=WBT_wbiFilename  wbiList=WBT_wbiList
  DotJ Nu3 : WBToolboxLibrary/wholeBodyModel/Jacobians/DotJ Nu  frameName='r_sole'  robotName=WBT_robotName  localName=WBT_modelName  wbiFile=WBT_wbiFilename  wbiList=WBT_wbiList
  Jacobian : WBToolboxLibrary/wholeBodyModel/Jacobians/Jacobian  frameName='com'  robotName=WBT_robotName  localName=WBT_modelName  wbiFile=WBT_wbiFilename  wbiList=WBT_wbiList
  Jacobian1 : WBToolboxLibrary/wholeBodyModel/Jacobians/Jacobian  frameName='root_link'  robotName=WBT_robotName  localName=WBT_modelName  wbiFile=WBT_wbiFilename  wbiList=WBT_wbiList
  Jacobian2 : WBToolboxLibrary/wholeBodyModel/Jacobians/Jacobian  frameName='l_sole'  robotName=WBT_robotName  localName=WBT_modelName  wbiFile=WBT_wbiFilename  wbiList=WBT_wbiList
  Jacobian3 : WBToolboxLibrary/wholeBodyModel/Jacobians/Jacobian  frameName='r_sole'  robotName=WBT_robotName  localName=WBT_modelName  wbiFile=WBT_wbiFilename  wbiList=WBT_wbiList
  Matrix Concatenate : Concatenate  NumInputs=4  Mode=Multidimensional array
  Matrix Concatenate1 : Concatenate  NumInputs=4  Mode=Multidimensional array
  Mux2 : Mux  Inputs=2
  Selector : Selector  InputPortWidth=6+ROBOT_DOF  IndexOptions=Index vector (dialog)  Indices=[1:6]  OutputSizes=1
  Selector1 : Selector  InputPortWidth=6+ROBOT_DOF  IndexOptions=Index vector (dialog)  Indices=[7:6+ROBOT_DOF]  OutputSizes=1
  Selector2 : Selector  NumberOfDimensions=2  InputPortWidth=6+ROBOT_DOF  IndexOptions=Index vector (dialog),Index vector (dialog)  Indices=[4:6],[1:6+ROBOT_DOF]  OutputSizes=1,1
  Selector3 : Selector  NumberOfDimensions=2  InputPortWidth=6+ROBOT_DOF  IndexOptions=Index vector (dialog),Index vector (dialog)  Indices=[1:3],[1:6+ROBOT_DOF]  OutputSizes=1,1
  Selector4 : Selector  InputPortWidth=6  IndexOptions=Index vector (dialog)  Indices=[1:3]  OutputSizes=1
  Selector5 : Selector  InputPortWidth=6  IndexOptions=Index vector (dialog)  Indices=[4:6]  OutputSizes=1
  baseVelocityFCN : MATLAB Function  TreatAsAtomicUnit=on
  Jc : Outport
  dJcNu : Outport  Port=2
  nu : Outport  Port=3
  wires:
  w_H_b/1 -> DotJ Nu1/1, DotJ Nu3/1, DotJ Nu2/1, DotJ Nu/1, Jacobian3/1, Jacobian2/1, Jacobian1/1, Jacobian/1
  qj/1 -> DotJ Nu3/2, DotJ Nu2/2, DotJ Nu1/2, DotJ Nu/2, Jacobian3/2, Jacobian2/2, Jacobian/2, Jacobian1/2
  Selector/1 -> DotJ Nu3/3, DotJ Nu2/3, DotJ Nu1/3, DotJ Nu/3
  Selector1/1 -> DotJ Nu1/4, DotJ Nu2/4, DotJ Nu3/4, DotJ Nu/4
  Mux2/1 -> nu/1, Selector1/1, Selector/1  "nu"
  Jacobian/1 -> Selector3/1
  Jacobian1/1 -> Selector2/1
  Selector3/1 -> Matrix Concatenate/1
  Selector2/1 -> Matrix Concatenate/2
  Matrix Concatenate/1 -> Jc/1
  DotJ Nu/1 -> Selector4/1
  DotJ Nu1/1 -> Selector5/1
  Selector4/1 -> Matrix Concatenate1/1
  Selector5/1 -> Matrix Concatenate1/2
  DotJ Nu2/1 -> Matrix Concatenate1/3
  DotJ Nu3/1 -> Matrix Concatenate1/4
  Matrix Concatenate1/1 -> dJcNu/1
  Jacobian3/1 -> baseVelocityFCN/2(JcRightFoot), Matrix Concatenate/4
  dqj/1 -> baseVelocityFCN/4(dqj), Mux2/2
  baseVelocityFCN/1(vb) -> Mux2/1
  feetConstraints/1 -> baseVelocityFCN/3(feetConstraints)
  Jacobian2/1 -> Matrix Concatenate/3, baseVelocityFCN/1(JcLeftFoot)

== system torqueBalancingSOT_logData/Dynamics, Kinematics, Jacobians/System Dynamics ==
  nu : Inport
  w_H_b : Inport  Port=2
  qj : Inport  Port=3
  Get Bias Forces : WBToolboxLibrary/wholeBodyModel/Dynamics/Get Bias Forces  robotName=WBT_robotName  localName=WBT_modelName  wbiFile=WBT_wbiFilename  wbiList=WBT_wbiList  explicitGravity=off
  Mass Matrix : WBToolboxLibrary/wholeBodyModel/Dynamics/Mass Matrix  robotName=WBT_robotName  localName=WBT_modelName  wbiFile=WBT_wbiFilename  wbiList=WBT_wbiList
  Selector : Selector  InputPortWidth=6+ROBOT_DOF  IndexOptions=Index vector (dialog)  Indices=[1:6]  OutputSizes=1
  Selector1 : Selector  InputPortWidth=6+ROBOT_DOF  IndexOptions=Index vector (dialog)  Indices=[7:6+ROBOT_DOF]  OutputSizes=1
  h : Outport
  M : Outport  Port=2
  wires:
  Selector/1 -> Get Bias Forces/3
  Selector1/1 -> Get Bias Forces/4
  w_H_b/1 -> Get Bias Forces/1, Mass Matrix/1
  Get Bias Forces/1 -> h/1
  Mass Matrix/1 -> M/1
  qj/1 -> Get Bias Forces/2, Mass Matrix/2
  nu/1 -> Selector1/1, Selector/1

== system torqueBalancingSOT_logData/Integration Based Inverse Kinematics/inverse kinematics integration ==
  qInit : Inport
  nuInit : Inport  Port=2
  dnuDes : Inport  Port=3
  Acceleration Integration : DiscreteIntegrator  InitialConditionSource=external  SampleTime=CONFIG.Ts  ICPrevOutput=DiscIntNeverNeededParam  ICPrevScaledInput=DiscIntNeverNeededParam
  Constant2 : Constant  Value=zeros(10,1)
  Constant3 : Constant  Value=zeros(10,1)
  Demux2 : Demux  Outputs=[7;ROBOT_DOF]
  Demux3 : Demux  Outputs=[6;ROBOT_DOF]
  Matrix Concatenate : Concatenate  NumInputs=3  Mode=Multidimensional array  ConcatenateDimension=2
  Mux3 : Mux  Inputs=2
  Mux4 : Mux  Inputs=2
  Mux5 : Mux  Inputs=2
  Terminator1 : Terminator
  Velocity Integration : DiscreteIntegrator  InitialConditionSource=external  SampleTime=CONFIG.Ts  ICPrevOutput=DiscIntNeverNeededParam  ICPrevScaledInput=DiscIntNeverNeededParam
  baseDerivative : MATLAB Function  TreatAsAtomicUnit=on
  rewrite the base pose as pos+quat : MATLAB Function  TreatAsAtomicUnit=on
  rewrite the base pose as transformation matrix : MATLAB Function  TreatAsAtomicUnit=on
  qDes : Outport
  nuDes : Outport  Port=2
  stateReferences : Outport  Port=3
  wires:
  nuInit/1 -> Acceleration Integration/2
  qInit/1 -> rewrite the base pose as pos+quat/1(qInitQuat)
  dnuDes/1 -> Mux5/2, Acceleration Integration/1
  Demux2/2 -> Terminator1/1
  Demux2/1 -> baseDerivative/1(basePose)
  Velocity Integration/1 -> Demux2/1, rewrite the base pose as transformation matrix/1(qDesQuat)
  Acceleration Integration/1 -> Mux4/2, Demux3/1, nuDes/1
  Demux3/1 -> baseDerivative/2(nuDes_base)
  baseDerivative/1(baseDer) -> Mux3/1
  Demux3/2 -> Mux3/2
  Mux3/1 -> Velocity Integration/1
  Matrix Concatenate/1 -> stateReferences/1
  rewrite the base pose as transformation matrix/1(qDes) -> Matrix Concatenate/1, qDes/1
  rewrite the base pose as pos+quat/1(qInit) -> Velocity Integration/2
  Constant2/1 -> Mux4/1
  Mux4/1 -> Matrix Concatenate/2
  Constant3/1 -> Mux5/1
  Mux5/1 -> Matrix Concatenate/3

== system torqueBalancingSOT_logData/Integration Based Inverse Kinematics/referenceAccelerations ==
  qDes : Inport
  nuDes : Inport  Port=2
  desCoMPosVelAcc : Inport  Port=3
  desTaskValues : Inport  Port=4
  desJointAngles : Inport  Port=5
  feetConstraints : Inport  Port=6
  impedances : Inport  Port=7
  dampings : Inport  Port=8
  PDgainsPos : Inport  Port=9
  PDgainsRot : Inport  Port=10
  Demux : Demux  Outputs=[16;ROBOT_DOF]
  Demux1 : Demux  Outputs=[6;ROBOT_DOF]
  Jacobians : Subsystem
  Kinematics : Subsystem
  Reshape : Reshape  OutputDimensionality=Customize  OutputDimensions=[4,4]
  Task and Joint Accelerations : Subsystem
  trajectoryGeneratorCoM2 : MATLAB Function  TreatAsAtomicUnit=on
  dnuDes : Outport
  wires:
  Demux/1 -> Reshape/1
  Demux1/2 -> Jacobians/4(jointVelocity), Task and Joint Accelerations/2(jointVelocities)
  qDes/1 -> Demux/1
  Reshape/1 -> Kinematics/1(w_H_b), Jacobians/1(w_H_b)
  Demux/2 -> Kinematics/2(JointAngles), Task and Joint Accelerations/4(jointAngles), Jacobians/2(JointAngles)
  feetConstraints/1 -> trajectoryGeneratorCoM2/5(constraints)
  trajectoryGeneratorCoM2/1(dnuDes) -> dnuDes/1
  nuDes/1 -> Demux1/1, Task and Joint Accelerations/3(nuDes)
  Jacobians/1(Jtask) -> Task and Joint Accelerations/1(Jtask), trajectoryGeneratorCoM2/1(Jtask)
  Jacobians/2(dJNu_task) -> trajectoryGeneratorCoM2/2(dJnuDes)
  Demux1/1 -> Jacobians/3(baseVelocity)
  desJointAngles/1 -> Task and Joint Accelerations/5(desJointAngles)
  Kinematics/3(w_H_lsole) -> Task and Joint Accelerations/8(w_H_lsole)
  Kinematics/4(w_H_rsole) -> Task and Joint Accelerations/9(w_H_rsole)
  Kinematics/1(CoMPos) -> Task and Joint Accelerations/6(CoMPos)
  Kinematics/2(w_R_root) -> Task and Joint Accelerations/7(W_R_root)
  desCoMPosVelAcc/1 -> Task and Joint Accelerations/10(desCoMPosVelAcc)
  desTaskValues/1 -> Task and Joint Accelerations/11(desTaskValues)
  Task and Joint Accelerations/2(jointsAccelerations) -> trajectoryGeneratorCoM2/4(jointDynamics)
  Task and Joint Accelerations/1(desTaskAcc) -> trajectoryGeneratorCoM2/3(taskAccelerations)
  impedances/1 -> Task and Joint Accelerations/12(impedances)
  dampings/1 -> Task and Joint Accelerations/13(dampings)
  PDgainsPos/1 -> Task and Joint Accelerations/14(PDgainsPos)
  PDgainsRot/1 -> Task and Joint Accelerations/15(PDgainsRot)

== system torqueBalancingSOT_logData/Visualize and log/Control gains ==
  state : Inport
  impedance : Inport  Port=2
  damping : Inport  Port=3
  Enable : EnablePort
  DoFs converter : WBToolboxLibrary/Utilities/DoFs converter  yarp2WBIOption=From WBI to YARP  robotName=WBT_robotName  localName=WBT_modelName  wbiFile=WBT_wbiFilename  wbiList=WBT_wbiList
  DoFs converter1 : WBToolboxLibrary/Utilities/DoFs converter  yarp2WBIOption=From WBI to YARP  robotName=WBT_robotName  localName=WBT_modelName  wbiFile=WBT_wbiFilename  wbiList=WBT_wbiList
  dampings : Scope  NumInputPorts=6
  impedances : Scope  NumInputPorts=6
  wires:
  DoFs converter/4 -> impedances/4  "left_leg"
  DoFs converter/5 -> impedances/5  "right_leg"
  DoFs converter/1 -> impedances/1  "torso"
  state/1 -> dampings/6, impedances/6  "state"
  DoFs converter1/3 -> dampings/3  "right_arm"
  damping/1 -> DoFs converter1/1
  impedance/1 -> DoFs converter/1
  DoFs converter1/1 -> dampings/1  "torso"
  DoFs converter/2 -> impedances/2  "left_arm"
  DoFs converter1/5 -> dampings/5  "right_leg"
  DoFs converter/3 -> impedances/3  "right_arm"
  DoFs converter1/2 -> dampings/2  "left_arm"
  DoFs converter1/4 -> dampings/4  "left_leg"

== system torqueBalancingSOT_logData/Visualize and log/Visualize eventual QP failures ==
  exitFlagQP : Inport
  state : Inport  Port=2
  Enable : EnablePort
  "QP status (0: no failure,  1: not using,  -1 internal error,  -2:  infeasible, -3:  unbounded) " : Scope  NumInputPorts=2
  wires:
  exitFlagQP/1 -> "QP status (0: no failure,  1: not using,  -1 internal error,  -2:  infeasible, -3:  unbounded) "/1  "exitFlagQP"
  state/1 -> "QP status (0: no failure,  1: not using,  -1 internal error,  -2:  infeasible, -3:  unbounded) "/2

== system torqueBalancingSOT_logData/Visualize and log/Visualize feet constraints ==
  wrench_leftFoot : Inport
  wrench_rightFoot : Inport  Port=2
  feetConstraints : Inport  Port=3
  state : Inport  Port=4
  Enable : EnablePort
  Feet Constraints : Scope  NumInputPorts=4
  wires:
  state/1 -> Feet Constraints/4  "state"
  feetConstraints/1 -> Feet Constraints/3  "feetConstraints"
  wrench_rightFoot/1 -> Feet Constraints/2  "wrench_rightFoot"
  wrench_leftFoot/1 -> Feet Constraints/1  "wrench_leftFoot"

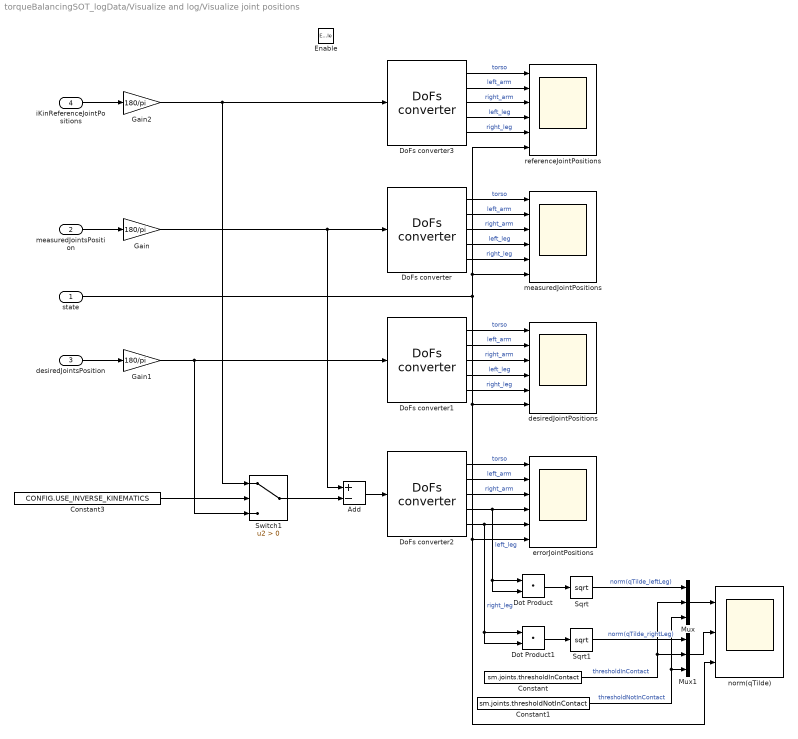
== system torqueBalancingSOT_logData/Visualize and log/Visualize joint positions ==
  state : Inport
  measuredJointsPosition : Inport  Port=2
  desiredJointsPosition : Inport  Port=3
  iKinReferenceJointPositions : Inport  Port=4
  Enable : EnablePort
  Add : Sum  Inputs=+-
  Constant : Constant  Value=sm.joints.thresholdInContact
  Constant1 : Constant  Value=sm.joints.thresholdNotInContact
  Constant3 : Constant  Value=CONFIG.USE_INVERSE_KINEMATICS
  DoFs converter{,1..3} (4 alike) : WBToolboxLibrary/Utilities/DoFs converter  yarp2WBIOption=From WBI to YARP  robotName=WBT_robotName  localName=WBT_modelName  wbiFile=WBT_wbiFilename  wbiList=WBT_wbiList
  Dot Product : DotProduct  InputSameDT=on  OutDataTypeStr=Inherit: Inherit via internal rule
  Dot Product1 : DotProduct  InputSameDT=on  OutDataTypeStr=Inherit: Inherit via internal rule
  Gain : Gain  Gain=180/pi
  Gain1 : Gain  Gain=180/pi
  Gain2 : Gain  Gain=180/pi
  Mux : Mux  Inputs=3
  Mux1 : Mux  Inputs=3
  Sqrt : Sqrt  SaturateOnIntegerOverflow=on
  Sqrt1 : Sqrt  SaturateOnIntegerOverflow=on
  Switch1 : Switch  Criteria=u2 > Threshold
  desiredJointPositions : Scope  NumInputPorts=6
  errorJointPositions : Scope  NumInputPorts=6
  measuredJointPositions : Scope  NumInputPorts=6
  norm(qTilde) : Scope  NumInputPorts=3
  referenceJointPositions : Scope  NumInputPorts=6
  wires:
  DoFs converter/5 -> measuredJointPositions/5  "right_leg"
  DoFs converter/4 -> measuredJointPositions/4  "left_leg"
  DoFs converter/2 -> measuredJointPositions/2  "left_arm"
  DoFs converter/1 -> measuredJointPositions/1  "torso"
  DoFs converter2/2 -> errorJointPositions/2  "left_arm"
  Gain1/1 -> DoFs converter1/1, Switch1/3
  DoFs converter2/1 -> errorJointPositions/1  "torso"
  desiredJointsPosition/1 -> Gain1/1
  measuredJointsPosition/1 -> Gain/1
  DoFs converter2/4 -> errorJointPositions/4, Dot Product/1, Dot Product/2  "left_leg"
  DoFs converter1/1 -> desiredJointPositions/1  "torso"
  DoFs converter1/3 -> desiredJointPositions/3  "right_arm"
  DoFs converter1/4 -> desiredJointPositions/4  "left_leg"
  Add/1 -> DoFs converter2/1
  Gain/1 -> Add/1, DoFs converter/1
  DoFs converter/3 -> measuredJointPositions/3  "right_arm"
  DoFs converter1/2 -> desiredJointPositions/2  "left_arm"
  DoFs converter2/3 -> errorJointPositions/3  "right_arm"
  DoFs converter2/5 -> errorJointPositions/5, Dot Product1/2, Dot Product1/1  "right_leg"
  DoFs converter1/5 -> desiredJointPositions/5  "right_leg"
  state/1 -> referenceJointPositions/6, measuredJointPositions/6, norm(qTilde)/3, errorJointPositions/6, desiredJointPositions/6
  Dot Product/1 -> Sqrt/1
  Dot Product1/1 -> Sqrt1/1
  Sqrt/1 -> Mux/1  "norm(qTilde_leftLeg)"
  Sqrt1/1 -> Mux1/1  "norm(qTilde_rightLeg)"
  Constant/1 -> Mux/2, Mux1/2  "thresholdInContact"
  Constant1/1 -> Mux1/3, Mux/3  "thresholdNotInContact"
  Mux/1 -> norm(qTilde)/1
  Mux1/1 -> norm(qTilde)/2
  DoFs converter3/5 -> referenceJointPositions/5  "right_leg"
  DoFs converter3/4 -> referenceJointPositions/4  "left_leg"
  DoFs converter3/2 -> referenceJointPositions/2  "left_arm"
  DoFs converter3/1 -> referenceJointPositions/1  "torso"
  DoFs converter3/3 -> referenceJointPositions/3  "right_arm"
  iKinReferenceJointPositions/1 -> Gain2/1
  Gain2/1 -> DoFs converter3/1, Switch1/1
  Switch1/1 -> Add/2
  Constant3/1 -> Switch1/2

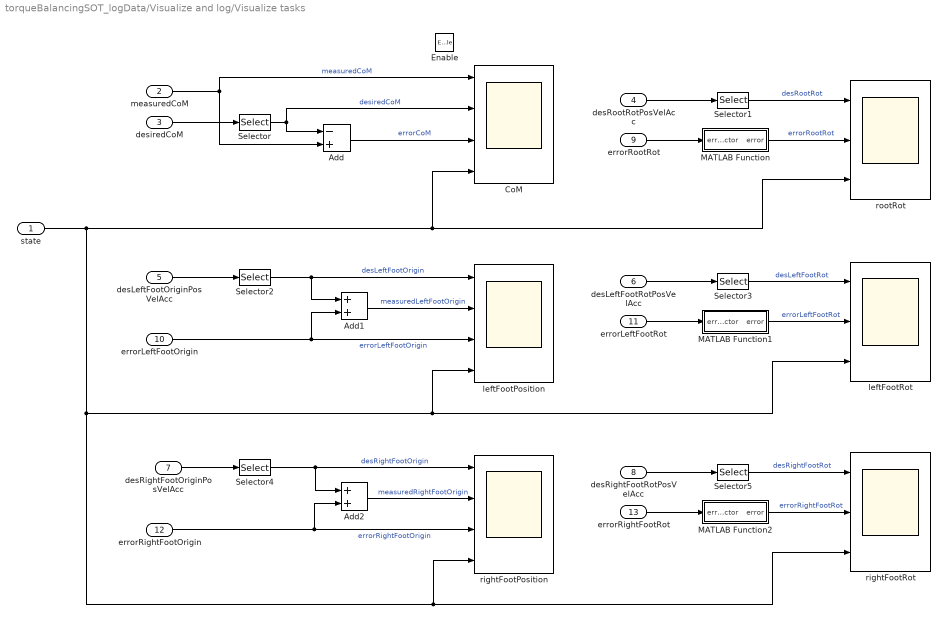
== system torqueBalancingSOT_logData/Visualize and log/Visualize tasks ==
  state : Inport
  measuredCoM : Inport  Port=2
  desiredCoM : Inport  Port=3
  desRootRotPosVelAcc : Inport  Port=4
  desLeftFootOriginPosVelAcc : Inport  Port=5
  desLeftFootRotPosVelAcc : Inport  Port=6
  desRightFootOriginPosVelAcc : Inport  Port=7
  desRightFootRotPosVelAcc : Inport  Port=8
  errorRootRot : Inport  Port=9
  errorLeftFootOrigin : Inport  Port=10
  errorLeftFootRot : Inport  Port=11
  errorRightFootOrigin : Inport  Port=12
  errorRightFootRot : Inport  Port=13
  Enable : EnablePort
  Add : Sum  Inputs=-+
  Add1 : Sum
  Add2 : Sum
  CoM : Scope  NumInputPorts=4
  MATLAB Function : MATLAB Function  TreatAsAtomicUnit=on
  MATLAB Function1 : MATLAB Function  TreatAsAtomicUnit=on
  MATLAB Function2 : MATLAB Function  TreatAsAtomicUnit=on
  Selector : Selector  NumberOfDimensions=2  InputPortWidth=9  IndexOptions=Index vector (dialog),Index vector (dialog)  Indices=[1:3],1  OutputSizes=1,1
  Selector1 : Selector  NumberOfDimensions=2  InputPortWidth=9  IndexOptions=Index vector (dialog),Index vector (dialog)  Indices=[1:3],[1:3]  OutputSizes=1,1
  Selector2 : Selector  NumberOfDimensions=2  InputPortWidth=9  IndexOptions=Index vector (dialog),Index vector (dialog)  Indices=[1:3],1  OutputSizes=1,1
  Selector3 : Selector  NumberOfDimensions=2  InputPortWidth=9  IndexOptions=Index vector (dialog),Index vector (dialog)  Indices=[1:3],[1:3]  OutputSizes=1,1
  Selector4 : Selector  NumberOfDimensions=2  InputPortWidth=9  IndexOptions=Index vector (dialog),Index vector (dialog)  Indices=[1:3],1  OutputSizes=1,1
  Selector5 : Selector  NumberOfDimensions=2  InputPortWidth=9  IndexOptions=Index vector (dialog),Index vector (dialog)  Indices=[1:3],[1:3]  OutputSizes=1,1
  leftFootPosition : Scope  NumInputPorts=4
  leftFootRot : Scope  NumInputPorts=3
  rightFootPosition : Scope  NumInputPorts=4
  rightFootRot : Scope  NumInputPorts=3
  rootRot : Scope  NumInputPorts=3
  wires:
  Selector/1 -> Add/1, CoM/2  "desiredCoM"
  Add/1 -> CoM/3  "errorCoM"
  desiredCoM/1 -> Selector/1
  state/1 -> rootRot/3, CoM/4, rightFootRot/3, rightFootPosition/4, leftFootPosition/4, leftFootRot/3
  measuredCoM/1 -> Add/2, CoM/1  "measuredCoM"
  desLeftFootOriginPosVelAcc/1 -> Selector2/1
  desRightFootOriginPosVelAcc/1 -> Selector4/1
  errorLeftFootOrigin/1 -> Add1/2, leftFootPosition/3  "errorLeftFootOrigin"
  errorRightFootOrigin/1 -> Add2/2, rightFootPosition/3  "errorRightFootOrigin"
  Selector2/1 -> Add1/1, leftFootPosition/1  "desLeftFootOrigin"
  Add1/1 -> leftFootPosition/2  "measuredLeftFootOrigin"
  Selector4/1 -> Add2/1, rightFootPosition/1  "desRightFootOrigin"
  Add2/1 -> rightFootPosition/2  "measuredRightFootOrigin"
  errorRootRot/1 -> MATLAB Function/1(errorVector)
  desRootRotPosVelAcc/1 -> Selector1/1
  desLeftFootRotPosVelAcc/1 -> Selector3/1
  errorLeftFootRot/1 -> MATLAB Function1/1(errorVector)
  desRightFootRotPosVelAcc/1 -> Selector5/1
  errorRightFootRot/1 -> MATLAB Function2/1(errorVector)
  MATLAB Function/1(error) -> rootRot/2  "errorRootRot"
  Selector1/1 -> rootRot/1  "desRootRot"
  Selector3/1 -> leftFootRot/1  "desLeftFootRot"
  MATLAB Function1/1(error) -> leftFootRot/2  "errorLeftFootRot"
  Selector5/1 -> rightFootRot/1  "desRightFootRot"
  MATLAB Function2/1(error) -> rightFootRot/2  "errorRightFootRot"
